simulink model "simulink_model_advanced_closed_loop"  (R2021a)
settings: Solver=VariableStepAuto  StartTime=0.0  StopTime=10  RelTol=1e-3
values from neighbouring files (symbols this model uses):
  N = 50    [main_race_car_ocp.m]
  nx = length(model.x)    [main_race_car_ocp.m]
settings Model: Creator=oj  LastModifiedBy=apl
settings SolverCC: AlgebraicLoopSolver=TrustRegion
settings DebuggingCC: SFMachineParentedDataDiag=warning
settings SFSimCC: CustomCodeUndefinedFunction=UseInterfaceOnly

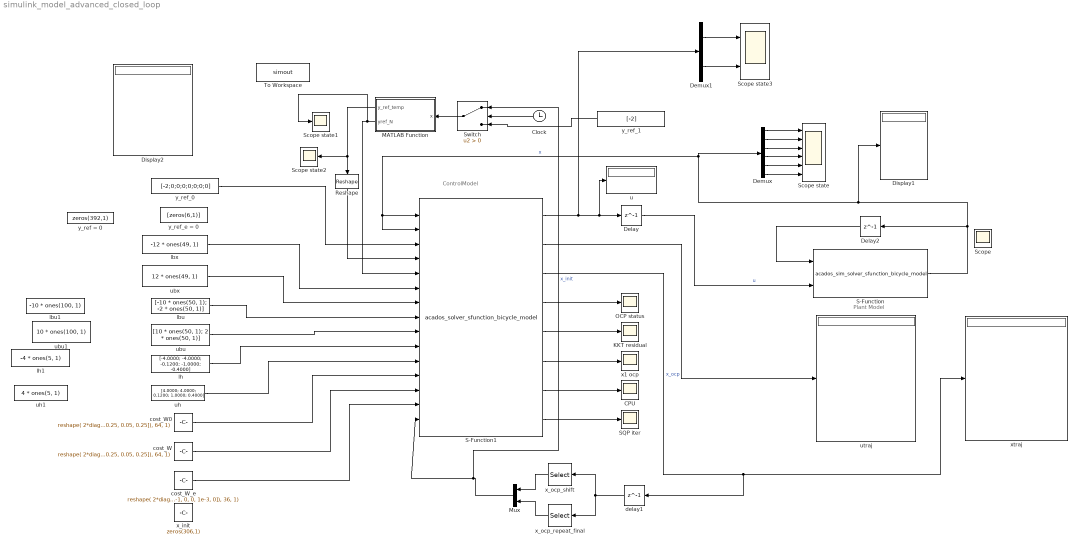
== system simulink_model_advanced_closed_loop ==
  note: ControlModel
  note: Plant Model
  CPU : Scope
      settings: Description=status
  Clock : Clock
  Delay : Delay  DelayLength=1  InitialCondition=0
  Delay2 : Delay  DelayLength=1  InitialCondition=[1 1 1 1 1 1]
  Demux : Demux  Outputs=6
  Demux1 : Demux  Outputs=2
  Display1 : Display
  Display2 : Display
  KKT residual : Scope
      settings: Description=status
  MATLAB Function : MATLAB Function  TreatAsAtomicUnit=on
  Mux : Mux  Inputs=2
  OCP status : Scope
      settings: Description=status
  Reshape : Reshape  OutputDimensionality=Customize  OutputDimensions=[392,1]
  S-Function : S-Function  FunctionName=acados_sim_solver_sfunction_bicycle_model  SFunctionDeploymentMode=off  EnableBusSupport=off
  S-Function1 : S-Function  FunctionName=acados_solver_sfunction_bicycle_model  SFunctionDeploymentMode=off  EnableBusSupport=off
  SQP iter : Scope
      settings: Description=status
  Scope state : Scope  NumInputPorts=6
  Scope state1 : Scope
  Scope state2 : Scope
  Scope state3 : Scope  NumInputPorts=2
  Switch : Switch  Criteria=u2 > Threshold
  To Workspace : ToWorkspace  VariableName=simout  SaveFormat=Structure With Time  SampleTime=-1
  cost_W : Constant  Value=reshape( 2*diag([5, 0, 0, 0, 0.05, 0.25, 0.05, 0.25]), 64, 1)
  cost_W0 : Constant  Value=reshape( 2*diag([5, 0, 0, 0, 0.05, 0.25, 0.05, 0.25]), 64, 1)
  cost_W_e : Constant  Value=reshape( 2*diag([1e-1, 2e-1, 0, 0, 1e-3, 0]), 36, 1)
  delay1 : Delay  DelayLength=1  InitialCondition=zeros(nx*(N+1),1)
  lbu : Constant  Value=[-10 * ones(50, 1); -2 * ones(50, 1)]
  lbu1 : Constant  Value=-10 * ones(100, 1)
  lbx : Constant  Value=-12 * ones(49, 1)
  lh : Constant  Value="[-4.0000;   -4.0000;   -0.1200;   -1.0000;   -0.4000]"
  lh1 : Constant  Value=-4 * ones(5, 1)
  u : Display
  ubu : Constant  Value=[10 * ones(50, 1); 2 * ones(50, 1)]
  ubu1 : Constant  Value=10 * ones(100, 1)
  ubx : Constant  Value=12 * ones(49, 1)
  uh : Constant  Value="[4.0000;    4.0000;    0.1200;    1.0000;    0.4000]"
  uh1 : Constant  Value=4 * ones(5, 1)
  utraj : Display
  x1 ocp : Scope
      settings: Description=status
  x_init : Constant  Value=zeros(306,1)
  x_ocp_repeat_final : Selector  IndexMode=Zero-based  InputPortWidth=(N+1)*nx  IndexOptions=Starting index (dialog)  Indices=N*nx  OutputSizes=nx
  x_ocp_shift : Selector  IndexMode=Zero-based  InputPortWidth=(N+1)*nx  IndexOptions=Starting index (dialog)  Indices=nx  OutputSizes=N*nx
  xtraj : Display
  y_ref = 0 : Constant  Value=zeros(392,1)
  y_ref_0 : Constant  Value=[-2;0;0;0;0;0;0;0]
  y_ref_1 : Constant  Value=[-2]
  y_ref_e = 0 : Constant  Value=[zeros(6,1)]
  Scope : Scope
  wires:
  S-Function/1 -> Display1/1, Demux/1, S-Function1/2, S-Function1/1, Delay2/1  "x"
  S-Function1/1 -> Demux1/1, u/1, Delay/1
  S-Function1/4 -> OCP status/1
  S-Function1/5 -> KKT residual/1
  S-Function1/6 -> x1 ocp/1
  S-Function1/7 -> CPU/1
  MATLAB Function/2(yref_N) -> Scope state1/1, S-Function1/5
  lbu/1 -> S-Function1/8
  ubu/1 -> S-Function1/9
  Delay/1 -> S-Function/2  "u"
  Delay2/1 -> S-Function/1
  S-Function1/8 -> SQP iter/1
  cost_W0/1 -> S-Function1/12
  cost_W/1 -> S-Function1/13
  cost_W_e/1 -> S-Function1/14
  S-Function1/2 -> utraj/1
  uh/1 -> S-Function1/11
  lh/1 -> S-Function1/10
  ubx/1 -> S-Function1/7
  lbx/1 -> S-Function1/6
  x_ocp_repeat_final/1 -> Mux/2
  Mux/1 -> Switch/1, S-Function1/15  "x_init"
  delay1/1 -> x_ocp_shift/1, x_ocp_repeat_final/1
  x_ocp_shift/1 -> Mux/1
  S-Function1/3 -> delay1/1, xtraj/1  "x_ocp"
  y_ref_0/1 -> S-Function1/3
  MATLAB Function/1(y_ref_temp) -> Scope state2/1, Reshape/1
  Reshape/1 -> S-Function1/4
  Switch/1 -> MATLAB Function/1(x)
  Clock/1 -> Switch/2
  y_ref_1/1 -> Switch/3
  Demux/1 -> Scope state/1
  Demux/2 -> Scope state/2
  Demux/3 -> Scope state/3
  Demux/4 -> Scope state/4
  Demux/5 -> Scope state/5
  Demux/6 -> Scope state/6
  Demux1/1 -> Scope state3/1
  Demux1/2 -> Scope state3/2

== matlab function simulink_model_advanced_closed_loop/MATLAB Function ==
  data: x input; y_ref_temp output size=8, 49; yref_N output
function [y_ref_temp, yref_N]   = fcn(x)
% track_file = 'LMS_Track.txt';
% [Sref, ~, ~, ~, ~] = getTrack(track_file);


% y_ref = zeros(1,392);
y_ref_temp = zeros(8,49);

s0 = x(7);  % equivalant of s0 = x0(1); from race car example main.m file
sref_N = 3;  % reference for final reference progress
N = 50;

% update reference
sref = s0 + sref_N;

%% MY Code
% y_ref(1,1:8) = [s0 + (sref - s0) * 0 / N, 0, 0, 0, 0, 0, 0, 0];
% 
% for j = 9:8:(N-2)
%     %  yref values for the shooting nodes 1 to N-1 concatenated
%     y_ref(1,j:j+7) = [s0 + (sref - s0) * j / N, 0, 0, 0, 0, 0, 0, 0];
% %     yref = [s0 + (sref - s0) * j / N, 0, 0, 0, 0, 0, 0, 0];
%     % yref=[1,0,0,1,0,0,0,0]
% %     ocp.set('cost_y_ref', yref, j);
% end
% 
k=1;
for j = 0:(N-2)
    %  yref values for the shooting nodes 1 to N-1 concatenated
    y_ref_temp(:,k) = [s0 + (sref - s0) * j / N, 0, 0, 0, 0, 0, 0, 0];
    k=k+1;
%     yref = [s0 + (sref - s0) * j / N, 0, 0, 0, 0, 0, 0, 0];
    % yref=[1,0,0,1,0,0,0,0]
%     ocp.set('cost_y_ref', yref, j);
end


yref_N = [sref, 0, 0, 0, 0, 0];
% ocp.set('cost_y_ref_e', yref_N);

stop_flag = 0;


% check if one lap is done and break and remove entries beyond
if s0 > 8.7105 + 0.1
    stop_flag = 1;
end

%% Org Code
% for j = 0:(N-1)
%     yref_t = [s0 + (sref - s0) * j / N, 0, 0, 0, 0, 0, 0, 0];
%     % yref=[1,0,0,1,0,0,0,0]
%     ocp.set('cost_y_ref', yref_t, j);   
% end
% yref_N = [sref, 0, 0, 0, 0, 0];
% % yref_N=np.array([0,0,0,0,0,0])    
% ocp.set('cost_y_ref_e', yref_N);

% y = y';

% yref_ = yref(:);

%y = yref;
